simulink model "ENEL441LabFall2012_Demo"  (R2012b)
settings: Solver=ode45  StartTime=0.0  StopTime=2  RelTol=1e-3
settings Model: Creator=kyle  LastModifiedBy=kyle
settings DataIOCC: InspectSignalLogs=on

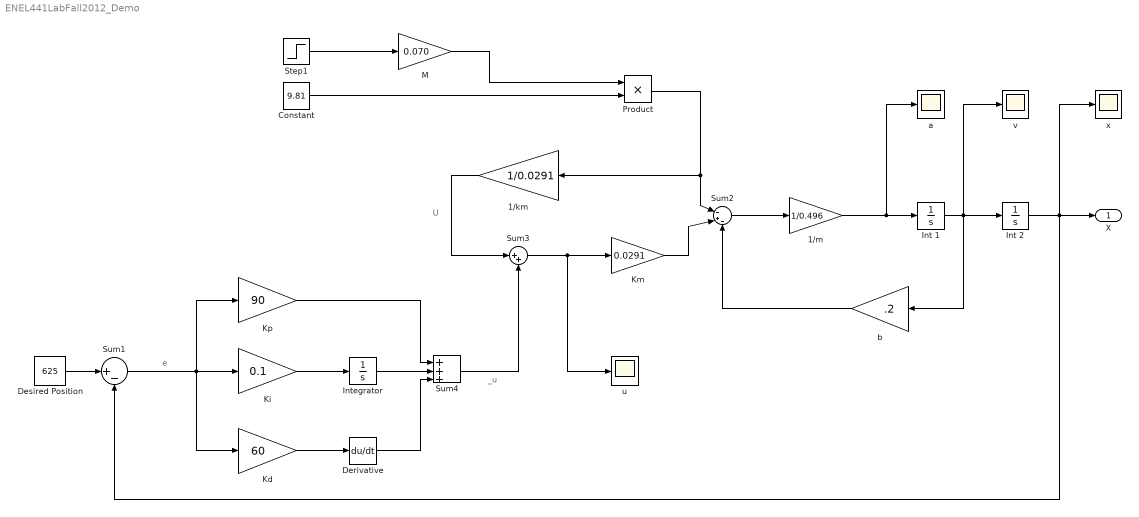
== system ENEL441LabFall2012_Demo ==
  note: e
  note: U
  note: _u
  1/km : Gain  Gain=1/0.0291
  1/m : Gain  Gain=1/0.496
  Constant : Constant  Value=9.81
  Derivative : Derivative
  Desired Position : Constant  Value=625
  Int 1 : Integrator
  Int 2 : Integrator
  Integrator : Integrator
  Kd : Gain  Gain=60
  Ki : Gain  Gain=0.1
  Km : Gain  Gain=0.0291
  Kp : Gain  Gain=90
  M : Gain  Gain=0.070
  Product : Product  RndMeth=Zero
  Step1 : Step  Time=0  SampleTime=0
  Sum1 : Sum  Inputs=|+-
  Sum2 : Sum  Inputs=|-+-
  Sum3 : Sum  Inputs=|++
  Sum4 : Sum  Inputs=|+++
  a : Scope
      settings: TimeRange=10  SaveName=ScopeData3
  b : Gain  Gain=.2
  u : Scope
      settings: TimeRange=500  SaveName=ScopeData5
  v : Scope
  x : Scope
      settings: TimeRange=20
  X : Outport
  wires:
  Km/1 -> Sum2/2
  b/1 -> Sum2/3
  Sum2/1 -> 1/m/1
  Int 1/1 -> b/1, v/1, Int 2/1
  Int 2/1 -> Sum1/2, X/1, x/1
  Constant/1 -> Product/2
  Step1/1 -> M/1
  Product/1 -> Sum2/1, 1/km/1
  M/1 -> Product/1
  1/m/1 -> a/1, Int 1/1
  1/km/1 -> Sum3/1
  Desired Position/1 -> Sum1/1
  Sum4/1 -> Sum3/2
  Sum3/1 -> Km/1, u/1
  Integrator/1 -> Sum4/2
  Sum1/1 -> Kp/1, Ki/1, Kd/1
  Kd/1 -> Derivative/1
  Ki/1 -> Integrator/1
  Derivative/1 -> Sum4/3
  Kp/1 -> Sum4/1
